simulink model "Bodes"  (R2018b)
settings: Solver=VariableStepAuto  StartTime=0.0  StopTime=10.0  RelTol=1e-3
libraries: slctrlblks x1
settings Model: Creator=xpess  LastModifiedBy=xpess

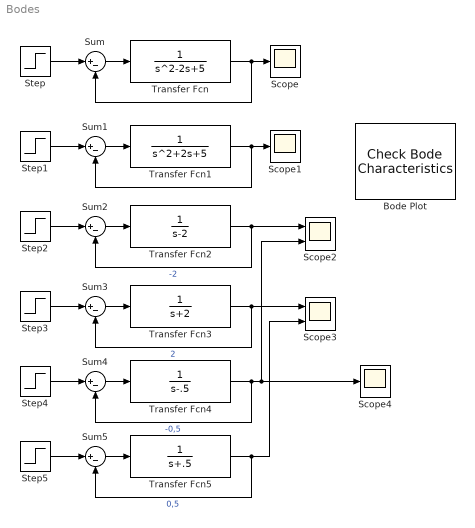
== system Bodes ==
  Bode Plot : slctrlblks/Model Verification/Check Bode  Characteristics  InstantiateOnLoad=on  SaveOperatingPoints=off  LinearizationIOs={'/Sum', 1, 'in', 'on', '';'/Sum1', 1, 'in', 'on', '';'/Sum2', 1, 'in', 'on', '';'/Sum3', 1, 'in', 'on', '';'/Sum4', 1, 'in', 'on', '';'/Sum5', 1, 'in', 'on', '';'/Transfer Fcn', 1, 'out', 'on', '';'/Transfer Fcn1', 1, 'out', 'on', '';'/Transfer Fcn2', 1, 'out', 'on', '';'/Transfer Fcn3', 1, 'out', 'on', '';'/Transfer Fcn4', 1, 'out', 'on', '';'/Transfer Fcn5', 1, 'out', 'on', ''}  LinearizeAt=SnapshotTimes  SnapshotTimes=[0]  TriggerType=rising  SampleTime=auto  RateConversionMethod=zoh  PreWarpFreq=10  UseExactDelayModel=off  UseFullBlockNameLabels=off  UseBusSignalLabels=off  enabled=on  stopWhenAssertionFail=off  export=off  ViewDlgPos=[1 41 1280 607.333333333333]  OpenViewOnLoad=off  LaunchViewOnOpen=off  FrequencyUnits=rad/s  MagnitudeUnits=dB  PhaseUnits=deg  TimeUnits=seconds  EnableUpperBound=off  UpperBoundFrequencies=[]  UpperBoundMagnitudes=[]  EnableLowerBound=off  LowerBoundFrequencies=[]  LowerBoundMagnitudes=[]
      settings: SourceProductName=Simulink Control Design
  Scope : Scope
  Scope1 : Scope
  Scope2 : Scope  NumInputPorts=2
  Scope3 : Scope  NumInputPorts=2
  Scope4 : Scope
  Step{,1..5} (6 alike) : Step  Time=0  SampleTime=0
  Sum{,1..5} (6 alike) : Sum  Inputs=|+-
  Transfer Fcn : TransferFcn  Denominator=[1 -2 5]
  Transfer Fcn1 : TransferFcn  Denominator=[1 2 5]
  Transfer Fcn2 : TransferFcn  Denominator=[1 -2]
  Transfer Fcn3 : TransferFcn  Denominator=[1 2]
  Transfer Fcn4 : TransferFcn  Denominator=[1 -.5]
  Transfer Fcn5 : TransferFcn  Denominator=[1 .5]
  wires:
  Step/1 -> Sum/1
  Sum/1 -> Transfer Fcn/1
  Transfer Fcn/1 -> Scope/1, Sum/2
  Step1/1 -> Sum1/1
  Transfer Fcn1/1 -> Scope1/1, Sum1/2
  Sum1/1 -> Transfer Fcn1/1
  Sum2/1 -> Transfer Fcn2/1
  Transfer Fcn2/1 -> Sum2/2, Scope2/1  "-2"
  Step2/1 -> Sum2/1
  Step3/1 -> Sum3/1
  Transfer Fcn3/1 -> Scope3/1, Sum3/2  "2"
  Sum3/1 -> Transfer Fcn3/1
  Sum4/1 -> Transfer Fcn4/1
  Transfer Fcn4/1 -> Sum4/2, Scope4/1, Scope2/2  "-0,5"
  Step4/1 -> Sum4/1
  Step5/1 -> Sum5/1
  Transfer Fcn5/1 -> Scope3/2, Sum5/2  "0,5"
  Sum5/1 -> Transfer Fcn5/1
